simulink model "PID_hm"  (R2020a)
settings: Solver=VariableStepAuto  StartTime=0.0  StopTime=10.0  RelTol=1e-3
settings Model: Creator=Finn  LastModifiedBy=Finn

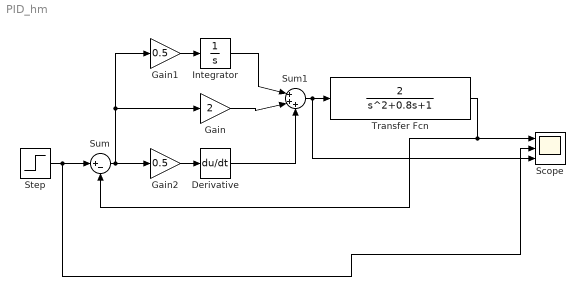
== system PID_hm ==
  Derivative : Derivative
  Gain : Gain  Gain=2
  Gain1 : Gain  Gain=0.5
  Gain2 : Gain  Gain=0.5
  Integrator : Integrator
  Scope : Scope  NumInputPorts=3
  Step : Step  Time=3  After=5  SampleTime=0
  Sum : Sum  Inputs=|+-
  Sum1 : Sum  Inputs=|+++
  Transfer Fcn : TransferFcn  Numerator=[2]  Denominator=[1,0.8,1]
  wires:
  Transfer Fcn/1 -> Sum/2, Scope/1
  Step/1 -> Scope/2, Sum/1
  Integrator/1 -> Sum1/1
  Derivative/1 -> Sum1/3
  Sum1/1 -> Scope/3, Transfer Fcn/1
  Gain/1 -> Sum1/2
  Gain1/1 -> Integrator/1
  Sum/1 -> Gain/1, Gain1/1, Gain2/1
  Gain2/1 -> Derivative/1
